simulink model "asdrd_ver2"  (R2018b)
settings: Solver=FixedStepAuto  StartTime=0.0  StopTime=200  FixedStep=1E-2  RelTol=1e-3
values from neighbouring files (symbols this model uses):
  A = [0  1; 0  0]    [data_ver2.mat]    (also in data_ver3.mat; just_running.m = [0,1;0,0])
  b = [0 1]    [data_ver2.mat]    (also in data_ver3.mat; just_running.m = [0;1])
  kT = block.DialogPrm(11).Data    [LeaderBlock.m]    (also in data_ver2.mat = [0.645779176886 6.55702927276]; data_ver3.mat = [0.22920630305 2.38997187052]; just_running.m = lqrd(A,b,Q,R,SumoTs))
  V = block.DialogPrm(12).Data    [LeaderBlock.m]    (also in data_ver2.mat = 0.645779176886; data_ver3.mat = 0.22920630305; just_running.m = -1./(cT*inv(A-b*kT)*b); tet_ver1.m = zeros(length(x),length(y)))
settings Model: Creator=HP  LastModifiedBy=HP

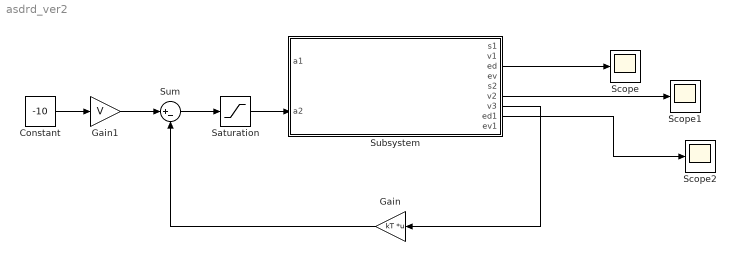
== system asdrd_ver2 ==
  Constant : Constant  Value=-10
  Gain : Gain  Gain=kT  Multiplication=Matrix(K*u)
  Gain1 : Gain  Gain=V
  Saturation : Saturate  UpperLimit=3  LowerLimit=-7
  Scope : Scope
  Scope1 : Scope
  Scope2 : Scope
  Subsystem : Subsystem
  Sum : Sum  Inputs=|+-
  wires:
  Subsystem/7(v3) -> Gain/1
  Constant/1 -> Gain1/1
  Sum/1 -> Saturation/1
  Gain1/1 -> Sum/1
  Gain/1 -> Sum/2
  Saturation/1 -> Subsystem/2(a2)
  Subsystem/3(ed) -> Scope/1
  Subsystem/6(v2) -> Scope1/1
  Subsystem/8(ed1) -> Scope2/1

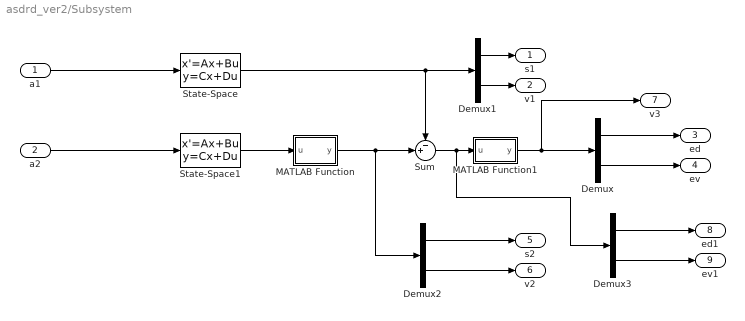
== system asdrd_ver2/Subsystem ==
  a1 : Inport
  a2 : Inport  Port=2
  Demux{,1..3} (4 alike) : Demux  Outputs=2
  MATLAB Function : MATLAB Function  TreatAsAtomicUnit=on
  MATLAB Function1 : MATLAB Function  TreatAsAtomicUnit=on
  State-Space : StateSpace  A=A  B=b  C=eye(2)  D=zeros(2,1)  InitialCondition=[0;20]
  State-Space1 : StateSpace  A=A  B=b  C=eye(2)  D=zeros(2,1)  InitialCondition=[-100;27]
  Sum : Sum  Inputs=-+|
  s1 : Outport
  v1 : Outport  Port=2
  ed : Outport  Port=3
  ev : Outport  Port=4
  s2 : Outport  Port=5
  v2 : Outport  Port=6
  v3 : Outport  Port=7
  ed1 : Outport  Port=8
  ev1 : Outport  Port=9
  wires:
  MATLAB Function/1(y) -> Demux2/1, Sum/2
  State-Space/1 -> Demux1/1, Sum/1
  State-Space1/1 -> MATLAB Function/1(u)
  a1/1 -> State-Space/1
  a2/1 -> State-Space1/1
  Sum/1 -> Demux3/1, MATLAB Function1/1(u)
  Demux/1 -> ed/1
  Demux/2 -> ev/1
  Demux1/1 -> s1/1
  Demux1/2 -> v1/1
  Demux2/1 -> s2/1
  Demux2/2 -> v2/1
  MATLAB Function1/1(y) -> v3/1, Demux/1
  Demux3/2 -> ev1/1
  Demux3/1 -> ed1/1

== matlab function asdrd_ver2/Subsystem/MATLAB Function1 ==
  data: u input; y output
function y = fcn(u)
y = [u(1);u(2)];
% if u(1) >= -4
%     y(1) = -4;
% else
%     y(1) = u(1);
% end

== matlab function asdrd_ver2/Subsystem/MATLAB Function ==
  data: u input; y output
function y = fcn(u)
y = [0;0]
if u(2) >= 25
    y(2) = 25;
    y(1) = u(1);
elseif u(2) <= 15
    y(2) = 15;
    y(1) = u(1);
else
    y(2) = u(2);
    y(1) = u(1);
end
